simulink model "mixTest123"  (R2020a)
settings: Solver=VariableStepAuto  StartTime=0.0  StopTime=1000  FixedStep=0.05  RelTol=1e-3
InitFcn:
  | data_current
values from neighbouring files (symbols this model uses):
  a1 = rho * D^4 * alpha1    (= 0.000388302366464)    [data_current.m]    (also in main_init.m)
  a2 = -rho * D^3 * alpha2 * (1 - omega)    (= 0.0037030698432)    [data_current.m]    (also in main_init.m)
  ag = [Ax Ay Az]'    [init_modello.m]
  alpha1 = 0.0113    [data_current.m]    (also in main_init.m)
  alpha2 = -0.0091    [data_current.m]    (also in main_init.m)
  areaOfInterestCorner = [42.317744;10.915136; 0]    [init_controllo.m]    (also in missionA.m = [42.317744)
  bg = [Bx By Bz]'    [init_modello.m]
  cd_pitch = 0.7    [init_modello.m]
  cd_roll = 0.04    [init_modello.m]
  cd_x = 0.4    [init_modello.m]
  cd_y = 1    [init_modello.m]
  cd_yaw = 0.7    [init_modello.m]
  cd_z = 1    [init_modello.m]
  cg = [Cx Cy Cz]'    [init_modello.m]
  D = 0.076    [data_current.m]    (also in main_init.m)
  dead_zone_limit = 31.5    [data_current.m]    (also in main_init.m)
  dg = [Dx Dy Dz]'    [init_modello.m]
  eg = [Ex Ey Ez]'    [init_modello.m]
  fg = [Fx Fy Fz]'    [init_modello.m]
  g = 9.81    [init_modello.m]
  galleggiamento = 66.5386    [init_controllo.m]
  gg = [Gx Gy Gz]'    [init_modello.m]
  H0 = 0    [init_modello.m]
  init_position = [pointP(1),pointP(2),0.15,0,0,deg2rad(angle)]'    [appunti.m]    (also in init_modello.m = [pointP(1),pointP(2),0.15,0,0,deg2rad(alpha)]')
  init_velocity = [0 0 0 0 0 0]'    [init_modello.m]
  Ixx = 0.93304097392    [init_modello.m]
  Ixy = 0    [init_modello.m]
  Ixz = 0    [init_modello.m]
  Iyy = 25.58745481378    (= 25.5874548138)    [init_modello.m]
  Iyz = 0    [init_modello.m]
  Izz = 25.58745481378    (= 25.5874548138)    [init_modello.m]
  K_i_heave_div = 20    [init_controllo.m]
  K_i_heave_pos = 1    [init_controllo.m]
  K_i_heave_surf = 20    [init_controllo.m]
  K_i_heave_trans = 5    [init_controllo.m]
  K_i_heave_turn = 5    [init_controllo.m]
  K_i_pitch_div = 0    [init_controllo.m]
  K_i_pitch_pos = 0.1*0    (= 0)    [init_controllo.m]
  K_i_pitch_surf = 0    [init_controllo.m]
  K_i_pitch_trans = 0    [init_controllo.m]
  K_i_pitch_turn = 0    [init_controllo.m]
  K_i_roll_div = 0    [init_controllo.m]
  K_i_roll_pos = 0.1*0    (= 0)    [init_controllo.m]
  K_i_roll_surf = 1    [init_controllo.m]
  K_i_roll_trans = 0    [init_controllo.m]
  K_i_roll_turn = 0    [init_controllo.m]
  K_i_surge_div = 3    [init_controllo.m]
  K_i_surge_pos = 0.1679*30    (= 5.037)    [init_controllo.m]
  K_i_surge_surf = 3    [init_controllo.m]
  K_i_surge_trans = 0.1679*15    (= 2.5185)    [init_controllo.m]
  K_i_surge_turn = 0.1679*60    (= 10.074)    [init_controllo.m]
  K_i_sway_div = 6    [init_controllo.m]
  K_i_sway_pos = 5    [init_controllo.m]
  K_i_sway_surf = 3    [init_controllo.m]
  K_i_sway_trans = 2    [init_controllo.m]
  K_i_sway_turn = 50    [init_controllo.m]
  K_i_yaw_div = 0    [init_controllo.m]
  K_i_yaw_pos = 1    [init_controllo.m]
  K_i_yaw_surf = 0    [init_controllo.m]
  K_i_yaw_trans = 20    [init_controllo.m]
  K_i_yaw_turn = 3    [init_controllo.m]
  K_p_heave_div = 200    [init_controllo.m]
  K_p_heave_pos = 320    [init_controllo.m]
  K_p_heave_surf = 200    [init_controllo.m]
  K_p_heave_trans = 170    [init_controllo.m]
  K_p_heave_turn = 170    [init_controllo.m]
  K_p_phi_div = 0.15    [init_controllo.m]
  K_p_phi_pos = 1*0.1    (= 0.1)    [init_controllo.m]
  K_p_phi_surf = 0.15    [init_controllo.m]
  K_p_phi_trans = 0.1    [init_controllo.m]
  K_p_phi_turn = 0.1    [init_controllo.m]
  K_p_pitch_div = 50    [init_controllo.m]
  K_p_pitch_pos = 25    [init_controllo.m]
  K_p_pitch_surf = 50    [init_controllo.m]
  K_p_pitch_trans = 25    [init_controllo.m]
  K_p_pitch_turn = 25    [init_controllo.m]
  K_p_psi_div = 0.3    [init_controllo.m]
  K_p_psi_pos = 0.25    [init_controllo.m]
  K_p_psi_surf = 0.3    [init_controllo.m]
  K_p_psi_trans = 0.2    [init_controllo.m]
  K_p_roll_div = 10    [init_controllo.m]
  K_p_roll_pos = 0.1*40    (= 4)    [init_controllo.m]
  K_p_roll_surf = 10    [init_controllo.m]
  K_p_roll_trans = 0.1*40    (= 4)    [init_controllo.m]
  K_p_roll_turn = 4    [init_controllo.m]
  K_p_surge_div = 80    [init_controllo.m]
  K_p_surge_pos = 13.7782*2.5    (= 34.4455)    [init_controllo.m]
  K_p_surge_surf = 80    [init_controllo.m]
  K_p_surge_trans = 20    [init_controllo.m]
  K_p_surge_turn = 150    [init_controllo.m]
  K_p_sway_div = 100    [init_controllo.m]
  K_p_sway_pos = 90    [init_controllo.m]
  K_p_sway_surf = 80    [init_controllo.m]
  K_p_sway_trans = 80    [init_controllo.m]
  K_p_sway_turn = 200    [init_controllo.m]
  K_p_th_div = 0.3    [init_controllo.m]
  K_p_th_pos = 0.1    [init_controllo.m]
  K_p_th_surf = 0.3    [init_controllo.m]
  K_p_th_trans = 0.1    [init_controllo.m]
  K_p_th_turn = 0.1    [init_controllo.m]
  K_p_x_div = 0.12    [init_controllo.m]
  K_p_x_pos = 0.12    [init_controllo.m]
  K_p_x_surf = 0.12    [init_controllo.m]
  K_p_y_div = 0.6    [init_controllo.m]
  K_p_y_pos = 0.34    [init_controllo.m]
  K_p_y_surf = 0.1    [init_controllo.m]
  K_p_y_trans = 0.3    [init_controllo.m]
  K_p_y_turn = 0.3    [init_controllo.m]
  K_p_yaw_div = 70    [init_controllo.m]
  K_p_yaw_pos = 20    [init_controllo.m]
  K_p_yaw_surf = 70    [init_controllo.m]
  K_p_yaw_trans = 160    [init_controllo.m]
  K_p_yaw_turn = 60    [init_controllo.m]
  K_p_z_div = 0.35    [init_controllo.m]
  K_p_z_pos = 0.2    [init_controllo.m]
  K_p_z_surf = 0.35    [init_controllo.m]
  K_p_z_trans = 0.10    (= 0.1)    [init_controllo.m]
  K_p_z_turn = 0.1    [init_controllo.m]
  Kadd = 0    [init_modello.m]
  m = 100    [init_modello.m]    (also in retta.m = p2-p1)
  ... (+29 more)
undefined symbols (not defined in the file or in its folder): DiscIntNeverNeededParam
libraries: simulink x4
(part 1 of 5)
settings Model: PauseTimes=1  PacingRate=5  Creator=User  LastModifiedBy=User

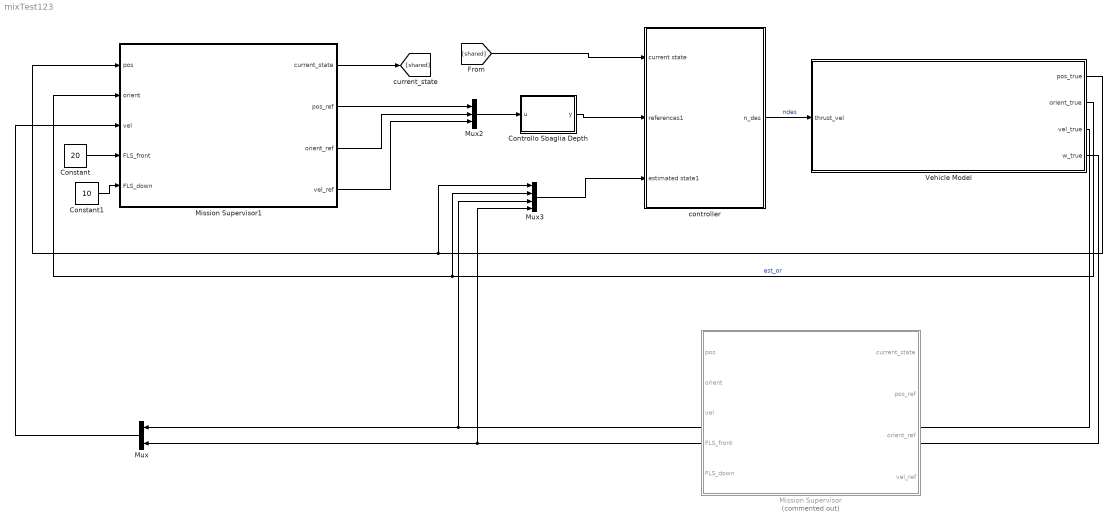
== system mixTest123 ==
  Constant : Constant  Value=20
  Constant1 : Constant  Value=10
  Controllo Sbaglia Depth : MATLAB Function  TreatAsAtomicUnit=on
  Mission Supervisor : Subsystem  Commented=on
  Mission Supervisor1 : Subsystem
  Mux : Mux  Inputs=2
  Mux2 : Mux  Inputs=3
  Mux3 : Mux
  Vehicle Model : Subsystem
  controller : Subsystem
  wires:
  Mission Supervisor1/1(current_state) -> [shared]
  Vehicle Model/3(vel_true) -> Mux3/3, Mux/1
  Vehicle Model/4(w_true) -> Mux3/4, Mux/2
  [shared] -> controller/1(current state)
  Mux2/1 -> Controllo Sbaglia Depth/1(u)
  Mux3/1 -> controller/3(estimated state1)
  controller/1(n_des) -> Vehicle Model/1(thrust_vel)  "ndes"
  Constant/1 -> Mission Supervisor1/4(FLS_front)
  Constant1/1 -> Mission Supervisor1/5(FLS_down)
  Controllo Sbaglia Depth/1(y) -> controller/2(references1)
  Vehicle Model/1(pos_true) -> Mission Supervisor1/1(pos), Mux3/1
  Mission Supervisor1/4(vel_ref) -> Mux2/3
  Vehicle Model/2(orient_true) -> Mission Supervisor1/2(orient), Mux3/2  "est_or"
  Mission Supervisor1/3(orient_ref) -> Mux2/2
  Mux/1 -> Mission Supervisor1/3(vel)
  Mission Supervisor1/2(pos_ref) -> Mux2/1

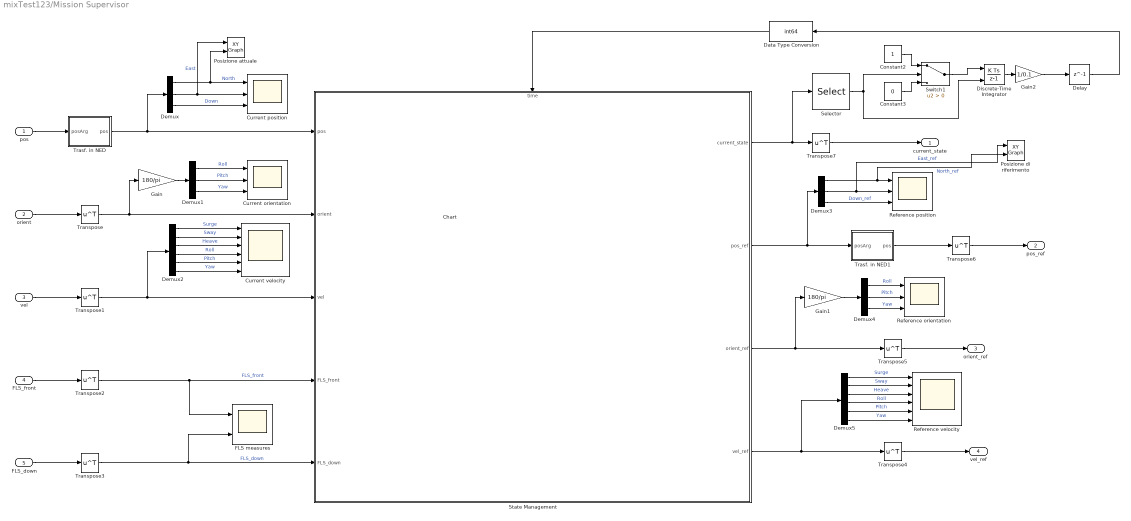
== system mixTest123/Mission Supervisor ==
  pos : Inport
  orient : Inport  Port=2  PortDimensions=[3 1]
  vel : Inport  Port=3  PortDimensions=[6 1]
  FLS_front : Inport  Port=4  PortDimensions=1
  FLS_down : Inport  Port=5  PortDimensions=1
  Chart : Stateflow chart  TreatAsAtomicUnit=on
  Constant2 : Constant
  Constant3 : Constant  Value=0
  Current orientation : Scope  NumInputPorts=3
  Current position : Scope  NumInputPorts=3
  Current velocity : Scope  NumInputPorts=6
  Data Type Conversion : DataTypeConversion  OutDataTypeStr=int64
  Delay : Delay  DelayLength=1  SampleTime=0.1
  Demux{,1,3..4} (4 alike) : Demux  Outputs=3
  Demux2 : Demux  Outputs=6
  Demux5 : Demux  Outputs=6
  Discrete-Time Integrator : DiscreteIntegrator  ExternalReset=falling  SampleTime=0.1  ICPrevOutput=DiscIntNeverNeededParam  ICPrevScaledInput=DiscIntNeverNeededParam
  FLS measures : Scope  NumInputPorts=2
  Gain : Gain  Gain=180/pi
  Gain1 : Gain  Gain=180/pi
  Gain2 : Gain  Gain=1/0.1
  Posizione attuale : simulink/Sinks/XY Graph  xmin=0  xmax=150  ymin=0  ymax=150  st=-1
  Posizione di riferimento : simulink/Sinks/XY Graph  xmin=0  xmax=150  ymin=0  ymax=150  st=-1
  Reference orientation : Scope  NumInputPorts=3
  Reference position : Scope  NumInputPorts=3
  Reference velocity : Scope  NumInputPorts=6
  Selector : Selector  InputPortWidth=8  IndexOptions=Index vector (dialog)  Indices=4  OutputSizes=1
  State Management : Stateflow chart  TreatAsAtomicUnit=on
      settings: PortSchema="{\"entries\":[{\"content\":{\"sides\":[{\"content\":{\"connectorIds\":[\"In1\",\"In2\",\"In3\",\"In4\",\"In5\"]},\"type\":\"ConnectorPlacement.EquallySpacedRectSide\",\"uuid\":\"b4d768e0-b402-4324-9a12-614211dc6b85\"},{\"content\":{\"connectorIds\":[\"Out1\",\"Out2\",\"Out3\",\"Out4\"],\"side\":\"RIGHT\"},\"type\":\"ConnectorPlacement.EquallySpacedRectSide\",\"uuid\":\"64a4c54a-28a4-456f-aa67-ad7da5d6855f\"},{\"content\":{\"connectorIds\":[\"In6\"],\"side\":\"TOP\"},\"type\":\"ConnectorPlacement.EquallySpacedRectSide\",\"uuid\":\"aacc81fd-f61d-4535-bc25-c566f9f9b0ba\"}]},\"type\":\"ConnectorPlacement.EquallySpacedConnector\",\"uuid\":\"1d5bfe1d-6e45-4fc8-afd6-fe82ea6d1d45\"}],\"packageUris\":[\"http://schema.mathworks.com/mf0/Connector/19700101\"],\"version\":\"1.0\"}"
  Switch1 : Switch  Criteria=u2 > Threshold
  Transpose{,1..7} (8 alike) : Math  Operator=transpose  SaturateOnIntegerOverflow=on
  Trasf. in NED : MATLAB Function  TreatAsAtomicUnit=on
  Trasf. in NED1 : MATLAB Function  TreatAsAtomicUnit=on
  current_state : Outport
  pos_ref : Outport  Port=2
  orient_ref : Outport  Port=3
  vel_ref : Outport  Port=4  PortDimensions=[6 1]
  wires:
  Transpose3/1 -> FLS measures/2, State Management/5(FLS_down)  "FLS_down"
  FLS_front/1 -> Transpose2/1
  Transpose5/1 -> orient_ref/1
  orient/1 -> Transpose/1
  vel/1 -> Transpose1/1
  Transpose4/1 -> vel_ref/1
  FLS_down/1 -> Transpose3/1
  Demux/1 -> Posizione attuale/2, Current position/1  "North"
  Demux/2 -> Posizione attuale/1, Current position/2  "East"
  Demux/3 -> Current position/3  "Down"
  Demux1/3 -> Current orientation/3  "Yaw"
  Demux1/2 -> Current orientation/2  "Pitch"
  Transpose/1 -> Gain/1, State Management/2(orient)
  Demux1/1 -> Current orientation/1  "Roll"
  Demux2/1 -> Current velocity/1  "Surge"
  Transpose1/1 -> Demux2/1, State Management/3(vel)
  Demux2/2 -> Current velocity/2  "Sway"
  Demux2/3 -> Current velocity/3  "Heave"
  Transpose2/1 -> FLS measures/1, State Management/4(FLS_front)  "FLS_front"
  Demux2/4 -> Current velocity/4  "Roll"
  Demux2/5 -> Current velocity/5  "Pitch"
  Demux2/6 -> Current velocity/6  "Yaw"
  Demux3/1 -> Posizione di riferimento/2, Reference position/1  "North_ref"
  Demux3/2 -> Posizione di riferimento/1, Reference position/2  "East_ref"
  Demux3/3 -> Reference position/3  "Down_ref"
  Demux4/1 -> Reference orientation/1  "Roll"
  State Management/3(orient_ref) -> Gain1/1, Transpose5/1
  Demux4/2 -> Reference orientation/2  "Pitch"
  Demux4/3 -> Reference orientation/3  "Yaw"
  Demux5/5 -> Reference velocity/5  "Pitch"
  Demux5/2 -> Reference velocity/2  "Sway"
  Demux5/1 -> Reference velocity/1  "Surge"
  Demux5/3 -> Reference velocity/3  "Heave"
  State Management/4(vel_ref) -> Demux5/1, Transpose4/1
  Demux5/4 -> Reference velocity/4  "Roll"
  Demux5/6 -> Reference velocity/6  "Yaw"
  pos/1 -> Trasf. in NED/1(posArg)
  State Management/2(pos_ref) -> Trasf. in NED1/1(posArg), Demux3/1
  Trasf. in NED1/1(pos) -> Transpose6/1
  Trasf. in NED/1(pos) -> Demux/1, State Management/1(pos)
  Transpose6/1 -> pos_ref/1
  Gain/1 -> Demux1/1
  Gain1/1 -> Demux4/1
  Transpose7/1 -> current_state/1
  Discrete-Time Integrator/1 -> Gain2/1
  Selector/1 -> Discrete-Time Integrator/2, Switch1/2
  Switch1/1 -> Discrete-Time Integrator/1
  Constant3/1 -> Switch1/3
  Constant2/1 -> Switch1/1
  Data Type Conversion/1 -> State Management/6(time)
  Gain2/1 -> Delay/1
  Delay/1 -> Data Type Conversion/1
  State Management/1(current_state) -> Selector/1, Transpose7/1

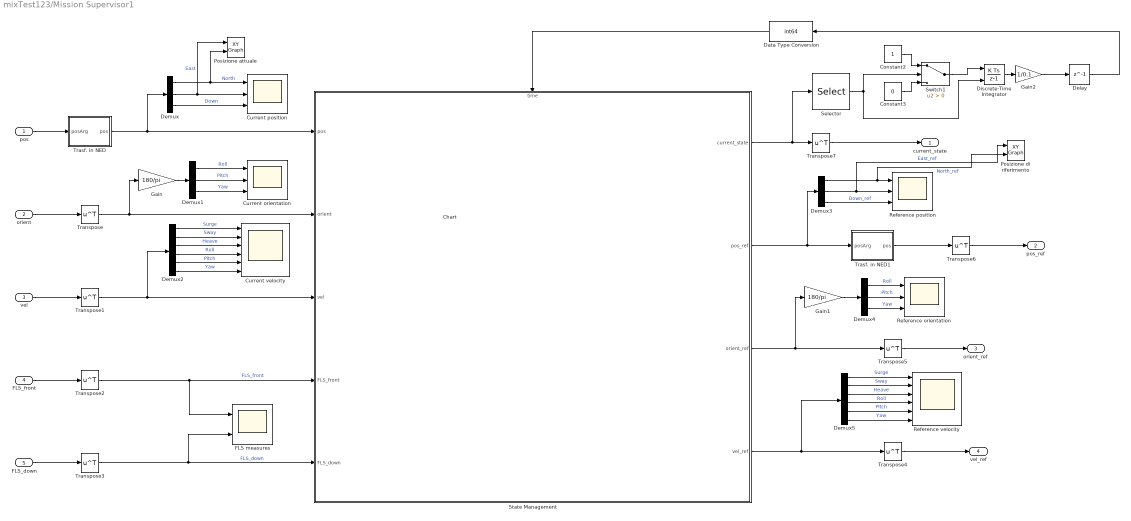
== system mixTest123/Mission Supervisor1 ==
  pos : Inport
  orient : Inport  Port=2  PortDimensions=[3 1]
  vel : Inport  Port=3  PortDimensions=[6 1]
  FLS_front : Inport  Port=4  PortDimensions=1
  FLS_down : Inport  Port=5  PortDimensions=1
  Chart : Stateflow chart  TreatAsAtomicUnit=on
  Constant2 : Constant
  Constant3 : Constant  Value=0
  Current orientation : Scope  NumInputPorts=3
  Current position : Scope  NumInputPorts=3
  Current velocity : Scope  NumInputPorts=6
  Data Type Conversion : DataTypeConversion  OutDataTypeStr=int64
  Delay : Delay  DelayLength=1  SampleTime=0.1
  Demux{,1,3..4} (4 alike) : Demux  Outputs=3
  Demux2 : Demux  Outputs=6
  Demux5 : Demux  Outputs=6
  Discrete-Time Integrator : DiscreteIntegrator  ExternalReset=falling  SampleTime=0.1  ICPrevOutput=DiscIntNeverNeededParam  ICPrevScaledInput=DiscIntNeverNeededParam
  FLS measures : Scope  NumInputPorts=2
  Gain : Gain  Gain=180/pi
  Gain1 : Gain  Gain=180/pi
  Gain2 : Gain  Gain=1/0.1
  Posizione attuale : simulink/Sinks/XY Graph  xmin=0  xmax=150  ymin=0  ymax=150  st=-1
  Posizione di riferimento : simulink/Sinks/XY Graph  xmin=0  xmax=150  ymin=0  ymax=150  st=-1
  Reference orientation : Scope  NumInputPorts=3
  Reference position : Scope  NumInputPorts=3
  Reference velocity : Scope  NumInputPorts=6
  Selector : Selector  InputPortWidth=8  IndexOptions=Index vector (dialog)  Indices=4  OutputSizes=1
  State Management : Stateflow chart  TreatAsAtomicUnit=on
      settings: PortSchema="{\"entries\":[{\"content\":{\"sides\":[{\"content\":{\"connectorIds\":[\"In1\",\"In2\",\"In3\",\"In4\",\"In5\"]},\"type\":\"ConnectorPlacement.EquallySpacedRectSide\",\"uuid\":\"b4d768e0-b402-4324-9a12-614211dc6b85\"},{\"content\":{\"connectorIds\":[\"Out1\",\"Out2\",\"Out3\",\"Out4\"],\"side\":\"RIGHT\"},\"type\":\"ConnectorPlacement.EquallySpacedRectSide\",\"uuid\":\"64a4c54a-28a4-456f-aa67-ad7da5d6855f\"},{\"content\":{\"connectorIds\":[\"In6\"],\"side\":\"TOP\"},\"type\":\"ConnectorPlacement.EquallySpacedRectSide\",\"uuid\":\"aacc81fd-f61d-4535-bc25-c566f9f9b0ba\"}]},\"type\":\"ConnectorPlacement.EquallySpacedConnector\",\"uuid\":\"1d5bfe1d-6e45-4fc8-afd6-fe82ea6d1d45\"}],\"packageUris\":[\"http://schema.mathworks.com/mf0/Connector/19700101\"],\"version\":\"1.0\"}"
  Switch1 : Switch  Criteria=u2 > Threshold
  Transpose{,1..7} (8 alike) : Math  Operator=transpose  SaturateOnIntegerOverflow=on
  Trasf. in NED : MATLAB Function  TreatAsAtomicUnit=on
  Trasf. in NED1 : MATLAB Function  TreatAsAtomicUnit=on
  current_state : Outport
  pos_ref : Outport  Port=2
  orient_ref : Outport  Port=3
  vel_ref : Outport  Port=4  PortDimensions=[6 1]
  wires:
  Transpose3/1 -> FLS measures/2, State Management/5(FLS_down)  "FLS_down"
  FLS_front/1 -> Transpose2/1
  Transpose5/1 -> orient_ref/1
  orient/1 -> Transpose/1
  vel/1 -> Transpose1/1
  Transpose4/1 -> vel_ref/1
  FLS_down/1 -> Transpose3/1
  Demux/1 -> Posizione attuale/2, Current position/1  "North"
  Demux/2 -> Posizione attuale/1, Current position/2  "East"
  Demux/3 -> Current position/3  "Down"
  Demux1/3 -> Current orientation/3  "Yaw"
  Demux1/2 -> Current orientation/2  "Pitch"
  Transpose/1 -> Gain/1, State Management/2(orient)
  Demux1/1 -> Current orientation/1  "Roll"
  Demux2/1 -> Current velocity/1  "Surge"
  Transpose1/1 -> Demux2/1, State Management/3(vel)
  Demux2/2 -> Current velocity/2  "Sway"
  Demux2/3 -> Current velocity/3  "Heave"
  Transpose2/1 -> FLS measures/1, State Management/4(FLS_front)  "FLS_front"
  Demux2/4 -> Current velocity/4  "Roll"
  Demux2/5 -> Current velocity/5  "Pitch"
  Demux2/6 -> Current velocity/6  "Yaw"
  Demux3/1 -> Posizione di riferimento/2, Reference position/1  "North_ref"
  Demux3/2 -> Posizione di riferimento/1, Reference position/2  "East_ref"
  Demux3/3 -> Reference position/3  "Down_ref"
  Demux4/1 -> Reference orientation/1  "Roll"
  State Management/3(orient_ref) -> Gain1/1, Transpose5/1
  Demux4/2 -> Reference orientation/2  "Pitch"
  Demux4/3 -> Reference orientation/3  "Yaw"
  Demux5/5 -> Reference velocity/5  "Pitch"
  Demux5/2 -> Reference velocity/2  "Sway"
  Demux5/1 -> Reference velocity/1  "Surge"
  Demux5/3 -> Reference velocity/3  "Heave"
  State Management/4(vel_ref) -> Demux5/1, Transpose4/1
  Demux5/4 -> Reference velocity/4  "Roll"
  Demux5/6 -> Reference velocity/6  "Yaw"
  pos/1 -> Trasf. in NED/1(posArg)
  State Management/2(pos_ref) -> Trasf. in NED1/1(posArg), Demux3/1
  Trasf. in NED1/1(pos) -> Transpose6/1
  Trasf. in NED/1(pos) -> Demux/1, State Management/1(pos)
  Transpose6/1 -> pos_ref/1
  Gain/1 -> Demux1/1
  Gain1/1 -> Demux4/1
  Transpose7/1 -> current_state/1
  Discrete-Time Integrator/1 -> Gain2/1
  Selector/1 -> Discrete-Time Integrator/2, Switch1/2
  Switch1/1 -> Discrete-Time Integrator/1
  Constant3/1 -> Switch1/3
  Constant2/1 -> Switch1/1
  Data Type Conversion/1 -> State Management/6(time)
  Gain2/1 -> Delay/1
  Delay/1 -> Data Type Conversion/1
  State Management/1(current_state) -> Selector/1, Transpose7/1

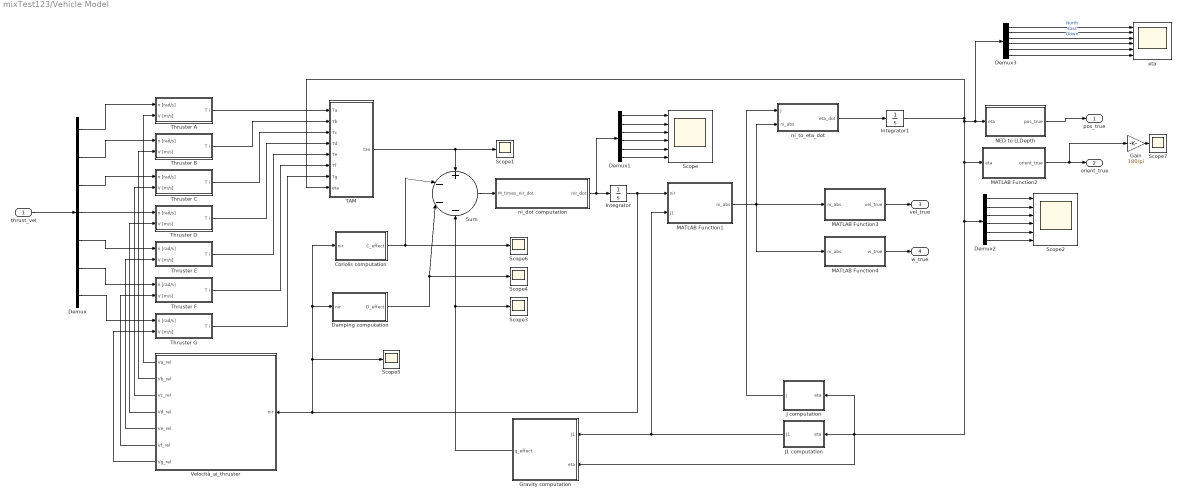
== system mixTest123/Vehicle Model ==
  thrust_vel : Inport
  Coriolis computation : MATLAB Function  TreatAsAtomicUnit=on
  Damping computation : MATLAB Function  TreatAsAtomicUnit=on
  Demux : Demux  Outputs=7
  Demux1 : Demux  Outputs=6
  Demux2 : Demux  Outputs=6
  Demux3 : Demux  Outputs=6
  Gain : Gain  Gain=180/pi
  Gravity computation : MATLAB Function  TreatAsAtomicUnit=on
  Integrator : Integrator  InitialCondition=init_velocity  ContinuousStateAttributes='velocity'
  Integrator1 : Integrator  InitialCondition=init_position  ContinuousStateAttributes='position'
  J computation : MATLAB Function  TreatAsAtomicUnit=on
  J1 computation : MATLAB Function  TreatAsAtomicUnit=on
  MATLAB Function1 : MATLAB Function  TreatAsAtomicUnit=on
  MATLAB Function2 : MATLAB Function  TreatAsAtomicUnit=on
  MATLAB Function3 : MATLAB Function  TreatAsAtomicUnit=on
  MATLAB Function4 : MATLAB Function  TreatAsAtomicUnit=on
  NED to LLDepth : MATLAB Function  TreatAsAtomicUnit=on
  Scope : Scope  NumInputPorts=6
  Scope{1,3..7} (6 alike) : Scope
  Scope2 : Scope  NumInputPorts=6
  Sum : Sum  Inputs=+---
  TAM : MATLAB Function
  Thruster A : Subsystem
  Thruster B : Subsystem
  Thruster C : Subsystem
  Thruster D : Subsystem
  Thruster E : Subsystem
  Thruster F : Subsystem
  Thruster G : Subsystem
  Velocità_ai_thruster : MATLAB Function  TreatAsAtomicUnit=on
  eta : Scope  NumInputPorts=6
  ni_dot computation : MATLAB Function  TreatAsAtomicUnit=on
  ni_to_eta_dot : MATLAB Function  TreatAsAtomicUnit=on
  pos_true : Outport
  orient_true : Outport  Port=2
  vel_true : Outport  Port=3
  w_true : Outport  Port=4
  wires:
  Demux/3 -> Thruster C/1(n [rad/s])
  Thruster A/1(T i) -> TAM/1(Ta)
  Thruster G/1(T i) -> TAM/7(Tg)
  Sum/1 -> ni_dot computation/1(M_times_nir_dot)
  Velocità_ai_thruster/7(Vg_rel) -> Thruster G/2(V [m/s])
  Velocità_ai_thruster/3(Vc_rel) -> Thruster C/2(V [m/s])
  Thruster C/1(T i) -> TAM/3(Tc)
  MATLAB Function3/1(vel_true) -> vel_true/1
  Gravity computation/1(g_effect) -> Sum/4, Scope3/1
  Demux/6 -> Thruster F/1(n [rad/s])
  MATLAB Function4/1(w_true) -> w_true/1
  J1 computation/1(J1) -> Gravity computation/1(J1), MATLAB Function1/2(J1)
  Thruster F/1(T i) -> TAM/6(Tf)
  Integrator/1 -> Scope5/1, Coriolis computation/1(nir), Damping computation/1(nir), Velocità_ai_thruster/1(nir), MATLAB Function1/1(nir)
  Velocità_ai_thruster/4(Vd_rel) -> Thruster D/2(V [m/s])
  Velocità_ai_thruster/6(Vf_rel) -> Thruster F/2(V [m/s])
  ni_dot computation/1(nir_dot) -> Demux1/1, Integrator/1
  Velocità_ai_thruster/2(Vb_rel) -> Thruster B/2(V [m/s])
  MATLAB Function1/1(ni_abs) -> ni_to_eta_dot/2(ni_abs), MATLAB Function3/1(ni_abs), MATLAB Function4/1(ni_abs)
  Velocità_ai_thruster/1(Va_rel) -> Thruster A/2(V [m/s])
  Demux/4 -> Thruster D/1(n [rad/s])
  Thruster E/1(T i) -> TAM/5(Te)
  Thruster B/1(T i) -> TAM/2(Tb)
  Demux/2 -> Thruster B/1(n [rad/s])
  TAM/1(tau) -> Sum/1, Scope1/1
  ni_to_eta_dot/1(eta_dot) -> Integrator1/1
  MATLAB Function2/1(orient_true) -> Gain/1, orient_true/1
  Demux/1 -> Thruster A/1(n [rad/s])
  Velocità_ai_thruster/5(Ve_rel) -> Thruster E/2(V [m/s])
  Demux/5 -> Thruster E/1(n [rad/s])
  NED to LLDepth/1(pos_true) -> pos_true/1
  Thruster D/1(T i) -> TAM/4(Td)
  J computation/1(J) -> ni_to_eta_dot/1(J)
  thrust_vel/1 -> Demux/1
  Demux/7 -> Thruster G/1(n [rad/s])
  Damping computation/1(D_effect) -> Sum/3, Scope4/1
  Coriolis computation/1(C_effect) -> Sum/2, Scope6/1
  Demux1/1 -> Scope/1
  Demux1/2 -> Scope/2
  Demux1/3 -> Scope/3
  Demux1/5 -> Scope/5
  Demux1/6 -> Scope/6
  Demux1/4 -> Scope/4
  Demux2/6 -> Scope2/6
  Demux2/5 -> Scope2/5
  Demux2/3 -> Scope2/3
  Demux2/2 -> Scope2/2
  Demux2/4 -> Scope2/4
  Demux2/1 -> Scope2/1
  Demux3/3 -> eta/3  "Down"
  Demux3/1 -> eta/1  "North"
  Demux3/2 -> eta/2  "East"
  Integrator1/1 -> TAM/8(eta), Demux3/1, NED to LLDepth/1(eta), J computation/1(eta), Gravity computation/2(eta), J1 computation/1(eta), Demux2/1, MATLAB Function2/1(eta)
  Demux3/4 -> eta/4
  Demux3/5 -> eta/5
  Demux3/6 -> eta/6
  Gain/1 -> Scope7/1

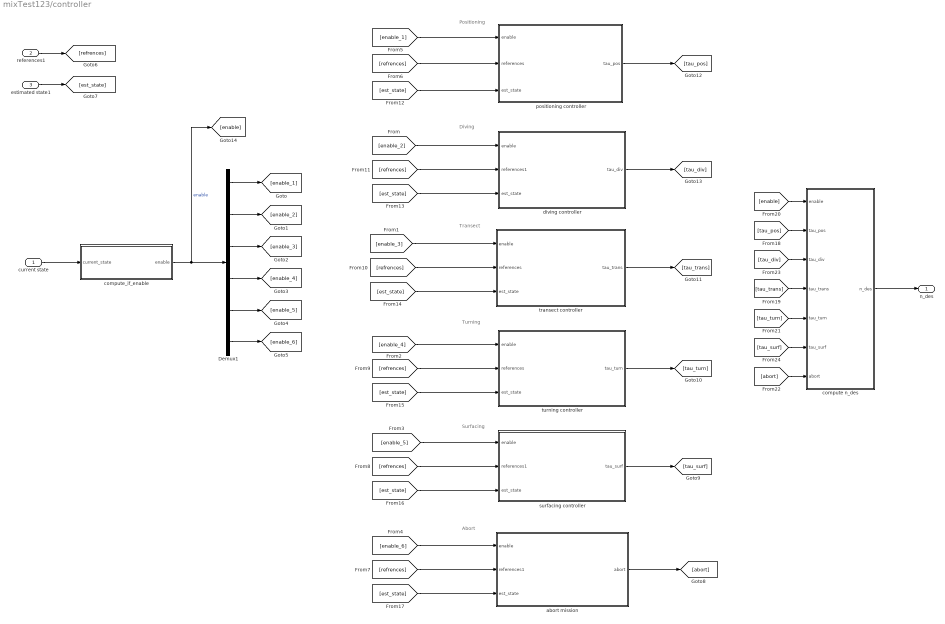
== system mixTest123/controller ==
  note: Diving
  note: Positioning
  note: Transect
  note: Abort
  note: Surfacing
  note: Turning
  current state : Inport
  references1 : Inport  Port=2
  estimated state1 : Inport  Port=3
  Demux1 : Demux  Outputs=6
  abort mission : Subsystem
  compute n_des : MATLAB Function  TreatAsAtomicUnit=on
  compute_if_enable : MATLAB Function  TreatAsAtomicUnit=on
  diving controller : Subsystem
  positioning controller : Subsystem
  surfacing controller : Subsystem
  transect controller : Subsystem
  turning controller : Subsystem
  n_des : Outport
  wires:
  [enable] -> compute n_des/1(enable)
  [enable_5] -> surfacing controller/1(enable)
  abort mission/1(abort) -> [abort]
  compute_if_enable/1(enable) -> [enable], Demux1/1  "enable"
  Demux1/3 -> [enable_3]
  Demux1/4 -> [enable_4]
  [tau_pos] -> compute n_des/2(tau_pos)
  [tau_surf] -> compute n_des/6(tau_surf)
  Demux1/5 -> [enable_5]
  Demux1/6 -> [enable_6]
  [refrences] -> diving controller/2(references1)
  references1/1 -> [refrences]
  turning controller/1(tau_turn) -> [tau_turn]
  [enable_2] -> diving controller/1(enable)
  [enable_4] -> turning controller/1(enable)
  [est_state] -> abort mission/3(est_state)
  current state/1 -> compute_if_enable/1(current_state)
  [tau_turn] -> compute n_des/5(tau_turn)
  [enable_1] -> positioning controller/1(enable)
  [refrences] -> abort mission/2(references1)
  Demux1/2 -> [enable_2]
  [est_state] -> turning controller/3(est_state)
  Demux1/1 -> [enable_1]
  [refrences] -> transect controller/2(references)
  diving controller/1(tau_div) -> [tau_div]
  [tau_trans] -> compute n_des/4(tau_trans)
  positioning controller/1(tau_pos) -> [tau_pos]
  [tau_div] -> compute n_des/3(tau_div)
  surfacing controller/1(tau_surf) -> [tau_surf]
  [abort] -> compute n_des/7(abort)
  [refrences] -> surfacing controller/2(references1)
  [enable_3] -> transect controller/1(enable)
  [refrences] -> positioning controller/2(references)
  [refrences] -> turning controller/2(references)
  [enable_6] -> abort mission/1(enable)
  estimated state1/1 -> [est_state]
  [est_state] -> positioning controller/3(est_state)
  [est_state] -> diving controller/3(est_state)
  transect controller/1(tau_trans) -> [tau_trans]
  [est_state] -> transect controller/3(est_state)
  [est_state] -> surfacing controller/3(est_state)
  compute n_des/1(n_des) -> n_des/1

== system mixTest123/Mission Supervisor/State Management/Movements.End ==
  f : TriggerPort  TriggerType=function-call  VariantControl=(inherit)
      settings: CopyFcn=Stateflow.SLINSF.SimulinkMan.removeBlockPreDeleteFcn  PreDeleteFcn=Stateflow.SLINSF.SimulinkMan.unsafePredeleteFcn
  Constant : Constant
  Stop Simulation : Stop
  wires:
  Constant/1 -> Stop Simulation/1

== system mixTest123/Mission Supervisor1/State Management/Movements.End ==
  f : TriggerPort  TriggerType=function-call  VariantControl=(inherit)
      settings: CopyFcn=Stateflow.SLINSF.SimulinkMan.removeBlockPreDeleteFcn  PreDeleteFcn=Stateflow.SLINSF.SimulinkMan.unsafePredeleteFcn
  Constant : Constant
  Stop Simulation : Stop
  wires:
  Constant/1 -> Stop Simulation/1

== system mixTest123/Vehicle Model/Thruster A ==
  note: n is the rotational speed of the thruster
      | V is the speed component of the water along the thruster axis
      |
      | n is saturated according to data
      | a dead zone is considered according to data
      | the thruster is characterised by 1st order dynamics (tau = 0.2s)
  n [rad/s] : Inport
  V [m/s] : Inport  Port=2
  Dead Zone : DeadZone  LowerValue=-dead_zone_limit  UpperValue=dead_zone_limit  SaturateOnIntegerOverflow=on
  MATLAB Function : MATLAB Function  TreatAsAtomicUnit=on
  Saturation : Saturate  UpperLimit=n_max  LowerLimit=-n_max
  Transfer Fcn : TransferFcn  Denominator=[0.2 1]
  T i : Outport
  wires:
  V [m/s]/1 -> MATLAB Function/2(V)
  Saturation/1 -> MATLAB Function/1(n)
  Transfer Fcn/1 -> Saturation/1
  Dead Zone/1 -> Transfer Fcn/1
  n [rad/s]/1 -> Dead Zone/1
  MATLAB Function/1(T) -> T i/1

== system mixTest123/Vehicle Model/Thruster B ==
  note: n is the rotational speed of the thruster
      | V is the speed component of the water along the thruster axis
      |
      | n is saturated according to data
      | a dead zone is considered according to data
      | the thruster is characterised by 1st order dynamics (tau = 0.2s)
  n [rad/s] : Inport
  V [m/s] : Inport  Port=2
  Dead Zone : DeadZone  LowerValue=-dead_zone_limit  UpperValue=dead_zone_limit  SaturateOnIntegerOverflow=on
  MATLAB Function : MATLAB Function  TreatAsAtomicUnit=on
  Saturation : Saturate  UpperLimit=n_max  LowerLimit=-n_max
  Transfer Fcn : TransferFcn  Denominator=[0.2 1]
  T i : Outport
  wires:
  MATLAB Function/1(T) -> T i/1
  n [rad/s]/1 -> Dead Zone/1
  Dead Zone/1 -> Transfer Fcn/1
  Transfer Fcn/1 -> Saturation/1
  Saturation/1 -> MATLAB Function/1(n)
  V [m/s]/1 -> MATLAB Function/2(V)

== system mixTest123/Vehicle Model/Thruster C ==
  note: n is the rotational speed of the thruster
      | V is the speed component of the water along the thruster axis
      |
      | n is saturated according to data
      | a dead zone is considered according to data
      | the thruster is characterised by 1st order dynamics (tau = 0.2s)
  n [rad/s] : Inport
  V [m/s] : Inport  Port=2
  Dead Zone : DeadZone  LowerValue=-dead_zone_limit  UpperValue=dead_zone_limit  SaturateOnIntegerOverflow=on
  MATLAB Function : MATLAB Function  TreatAsAtomicUnit=on
  Saturation : Saturate  UpperLimit=n_max  LowerLimit=-n_max
  Transfer Fcn : TransferFcn  Denominator=[0.2 1]
  T i : Outport
  wires:
  V [m/s]/1 -> MATLAB Function/2(V)
  Saturation/1 -> MATLAB Function/1(n)
  Transfer Fcn/1 -> Saturation/1
  Dead Zone/1 -> Transfer Fcn/1
  n [rad/s]/1 -> Dead Zone/1
  MATLAB Function/1(T) -> T i/1

== system mixTest123/Vehicle Model/Thruster D ==
  note: n is the rotational speed of the thruster
      | V is the speed component of the water along the thruster axis
      |
      | n is saturated according to data
      | a dead zone is considered according to data
      | the thruster is characterised by 1st order dynamics (tau = 0.2s)
  n [rad/s] : Inport
  V [m/s] : Inport  Port=2
  Dead Zone : DeadZone  LowerValue=-dead_zone_limit  UpperValue=dead_zone_limit  SaturateOnIntegerOverflow=on
  MATLAB Function : MATLAB Function  TreatAsAtomicUnit=on
  Saturation : Saturate  UpperLimit=n_max  LowerLimit=-n_max
  Transfer Fcn : TransferFcn  Denominator=[0.2 1]
  T i : Outport
  wires:
  MATLAB Function/1(T) -> T i/1
  n [rad/s]/1 -> Dead Zone/1
  Dead Zone/1 -> Transfer Fcn/1
  Transfer Fcn/1 -> Saturation/1
  Saturation/1 -> MATLAB Function/1(n)
  V [m/s]/1 -> MATLAB Function/2(V)

== system mixTest123/Vehicle Model/Thruster E ==
  note: n is the rotational speed of the thruster
      | V is the speed component of the water along the thruster axis
      |
      | n is saturated according to data
      | a dead zone is considered according to data
      | the thruster is characterised by 1st order dynamics (tau = 0.2s)
  n [rad/s] : Inport
  V [m/s] : Inport  Port=2
  Dead Zone : DeadZone  LowerValue=-dead_zone_limit  UpperValue=dead_zone_limit  SaturateOnIntegerOverflow=on
  MATLAB Function : MATLAB Function  TreatAsAtomicUnit=on
  Saturation : Saturate  UpperLimit=n_max  LowerLimit=-n_max
  Transfer Fcn : TransferFcn  Denominator=[0.2 1]
  T i : Outport
  wires:
  V [m/s]/1 -> MATLAB Function/2(V)
  Saturation/1 -> MATLAB Function/1(n)
  Transfer Fcn/1 -> Saturation/1
  Dead Zone/1 -> Transfer Fcn/1
  n [rad/s]/1 -> Dead Zone/1
  MATLAB Function/1(T) -> T i/1

== system mixTest123/Vehicle Model/Thruster F ==
  note: n is the rotational speed of the thruster
      | V is the speed component of the water along the thruster axis
      |
      | n is saturated according to data
      | a dead zone is considered according to data
      | the thruster is characterised by 1st order dynamics (tau = 0.2s)
  n [rad/s] : Inport
  V [m/s] : Inport  Port=2
  Dead Zone : DeadZone  LowerValue=-dead_zone_limit  UpperValue=dead_zone_limit  SaturateOnIntegerOverflow=on
  MATLAB Function : MATLAB Function  TreatAsAtomicUnit=on
  Saturation : Saturate  UpperLimit=n_max  LowerLimit=-n_max
  Transfer Fcn : TransferFcn  Denominator=[0.2 1]
  T i : Outport
  wires:
  MATLAB Function/1(T) -> T i/1
  n [rad/s]/1 -> Dead Zone/1
  Dead Zone/1 -> Transfer Fcn/1
  Transfer Fcn/1 -> Saturation/1
  Saturation/1 -> MATLAB Function/1(n)
  V [m/s]/1 -> MATLAB Function/2(V)

== system mixTest123/Vehicle Model/Thruster G ==
  note: n is the rotational speed of the thruster
      | V is the speed component of the water along the thruster axis
      |
      | n is saturated according to data
      | a dead zone is considered according to data
      | the thruster is characterised by 1st order dynamics (tau = 0.2s)
  n [rad/s] : Inport
  V [m/s] : Inport  Port=2
  Dead Zone : DeadZone  LowerValue=-dead_zone_limit  UpperValue=dead_zone_limit  SaturateOnIntegerOverflow=on
  MATLAB Function : MATLAB Function  TreatAsAtomicUnit=on
  Saturation : Saturate  UpperLimit=n_max  LowerLimit=-n_max
  Transfer Fcn : TransferFcn  Denominator=[0.2 1]
  T i : Outport
  wires:
  V [m/s]/1 -> MATLAB Function/2(V)
  Saturation/1 -> MATLAB Function/1(n)
  Transfer Fcn/1 -> Saturation/1
  Dead Zone/1 -> Transfer Fcn/1
  n [rad/s]/1 -> Dead Zone/1
  MATLAB Function/1(T) -> T i/1

== system mixTest123/controller/abort mission ==
  enable : Inport
  references1 : Inport  Port=2
  est_state : Inport  Port=3
  abort mission : MATLAB Function  TreatAsAtomicUnit=on
  abort : Outport
  wires:
  enable/1 -> abort mission/1(enable)
  references1/1 -> abort mission/2(ref)
  est_state/1 -> abort mission/3(est_meas)
  abort mission/1(abort) -> abort/1

== system mixTest123/controller/diving controller ==
  enable : Inport
  references1 : Inport  Port=2
  est_state : Inport  Port=3
  Mux : Mux  Inputs=6
  heave_controller : Subsystem
  pitch_controller : Subsystem
  roll_controller : Subsystem
  surge_controller : Subsystem
  sway_controller : Subsystem
  yaw_controller : Subsystem
  tau_div : Outport
  wires:
  sway_controller/1(Y) -> Mux/2  "Y"
  yaw_controller/1(N) -> Mux/6  "N"
  Mux/1 -> tau_div/1
  heave_controller/1(Z) -> Mux/3  "Z"
  references1/1 -> surge_controller/2(references), heave_controller/2(references), roll_controller/2(references), yaw_controller/2(references), pitch_controller/2(references), sway_controller/2(references)
  est_state/1 -> sway_controller/3("estimated measures "), heave_controller/3("estimated measures "), roll_controller/3("estimated measures "), yaw_controller/3("estimated measures "), pitch_controller/3("estimated measures "), surge_controller/3("estimated measures ")
  surge_controller/1(X) -> Mux/1  "X"
  roll_controller/1(K) -> Mux/4  "K"
  pitch_controller/1(M) -> Mux/5  "M"
  enable/1 -> sway_controller/1(enable), heave_controller/1(enable), yaw_controller/1(enable), pitch_controller/1(enable), roll_controller/1(enable), surge_controller/1(enable)

== system mixTest123/controller/positioning controller ==
  enable : Inport
  references : Inport  Port=2
  est_state : Inport  Port=3
  Mux : Mux  Inputs=6
  heave_controller : Subsystem
  pitch_controller : Subsystem
  roll_controller : Subsystem
  surge_controller : Subsystem
  sway_controller : Subsystem
  yaw_controller : Subsystem
  tau_pos : Outport
  wires:
  enable/1 -> sway_controller/1(enable), heave_controller/1(enable), yaw_controller/1(enable), pitch_controller/1(enable), roll_controller/1(enable), surge_controller/1(enable)
  yaw_controller/1(N) -> Mux/6  "N"
  references/1 -> surge_controller/2(references), heave_controller/2(references), roll_controller/2(references), yaw_controller/2(references), pitch_controller/2(references), sway_controller/2(references)
  pitch_controller/1(M) -> Mux/5  "M"
  est_state/1 -> sway_controller/3("estimated measures "), heave_controller/3("estimated measures "), roll_controller/3("estimated measures "), yaw_controller/3("estimated measures "), pitch_controller/3("estimated measures "), surge_controller/3("estimated measures ")
  surge_controller/1(X) -> Mux/1  "X"
  sway_controller/1(Y) -> Mux/2  "Y"
  roll_controller/1(K) -> Mux/4  "K"
  Mux/1 -> tau_pos/1
  heave_controller/1(Z) -> Mux/3  "Z"

== system mixTest123/controller/surfacing controller ==
  enable : Inport
  references1 : Inport  Port=2
  est_state : Inport  Port=3
  Mux : Mux  Inputs=6
  heave_controller : Subsystem
  pitch_controller : Subsystem
  roll_controller : Subsystem
  surge_controller : Subsystem
  sway_controller : Subsystem
  yaw_controller : Subsystem
  tau_surf : Outport
  wires:
  sway_controller/1(Y) -> Mux/2  "Y"
  yaw_controller/1(N) -> Mux/6  "N"
  Mux/1 -> tau_surf/1
  heave_controller/1(Z) -> Mux/3  "Z"
  references1/1 -> surge_controller/2(references), heave_controller/2(references), roll_controller/2(references), yaw_controller/2(references), pitch_controller/2(references), sway_controller/2(references)
  est_state/1 -> sway_controller/3("estimated measures "), heave_controller/3("estimated measures "), roll_controller/3("estimated measures "), yaw_controller/3("estimated measures "), pitch_controller/3("estimated measures "), surge_controller/3("estimated measures ")
  surge_controller/1(X) -> Mux/1  "X"
  roll_controller/1(K) -> Mux/4  "K"
  pitch_controller/1(M) -> Mux/5  "M"
  enable/1 -> sway_controller/1(enable), heave_controller/1(enable), yaw_controller/1(enable), pitch_controller/1(enable), roll_controller/1(enable), surge_controller/1(enable)

== system mixTest123/controller/transect controller ==
  enable : Inport
  references : Inport  Port=2
  est_state : Inport  Port=3
  Mux : Mux  Inputs=6
  heave_controller : Subsystem
  pitch_controller : Subsystem
  roll_controller : Subsystem
  surge_controller : Subsystem
  sway_controller : Subsystem
  yaw_controller : Subsystem
  tau_trans : Outport
  wires:
  sway_controller/1(Y) -> Mux/2  "Y"
  yaw_controller/1(N) -> Mux/6  "N"
  Mux/1 -> tau_trans/1
  heave_controller/1(Z) -> Mux/3  "Z"
  references/1 -> surge_controller/2(references), heave_controller/2(references), roll_controller/2(references), yaw_controller/2(references), pitch_controller/2(references), sway_controller/2(references)
  est_state/1 -> sway_controller/3("estimated measures "), heave_controller/3("estimated measures "), roll_controller/3("estimated measures "), yaw_controller/3("estimated measures "), pitch_controller/3("estimated measures "), surge_controller/3("estimated measures ")
  surge_controller/1(X) -> Mux/1  "X"
  roll_controller/1(K) -> Mux/4  "K"
  pitch_controller/1(M) -> Mux/5  "M"
  enable/1 -> sway_controller/1(enable), heave_controller/1(enable), yaw_controller/1(enable), pitch_controller/1(enable), roll_controller/1(enable), surge_controller/1(enable)

== system mixTest123/controller/turning controller ==
  enable : Inport
  references : Inport  Port=2
  est_state : Inport  Port=3
  Mux : Mux  Inputs=6
  heave_controller : Subsystem
  pitch_controller : Subsystem
  roll_controller : Subsystem
  surge_controller : Subsystem
  sway_controller : Subsystem
  yaw_controller : Subsystem
  tau_turn : Outport
  wires:
  sway_controller/1(Y) -> Mux/2  "Y"
  yaw_controller/1(N) -> Mux/6  "N"
  Mux/1 -> tau_turn/1
  heave_controller/1(Z) -> Mux/3  "Z"
  references/1 -> surge_controller/2(references), heave_controller/2(references), roll_controller/2(references), yaw_controller/2(references), pitch_controller/2(references), sway_controller/2(references)
  est_state/1 -> sway_controller/3("estimated measures "), heave_controller/3("estimated measures "), roll_controller/3("estimated measures "), yaw_controller/3("estimated measures "), pitch_controller/3("estimated measures "), surge_controller/3("estimated measures ")
  surge_controller/1(X) -> Mux/1  "X"
  roll_controller/1(K) -> Mux/4  "K"
  pitch_controller/1(M) -> Mux/5  "M"
  enable/1 -> sway_controller/1(enable), heave_controller/1(enable), yaw_controller/1(enable), pitch_controller/1(enable), roll_controller/1(enable), surge_controller/1(enable)

== system mixTest123/controller/diving controller/heave_controller ==
  enable : Inport
  references : Inport  Port=2
  "estimated measures " : Inport  Port=3
  Heave PID controller : Subsystem
  Z : Outport
  wires:
  Heave PID controller/1(Z) -> Z/1  "Z_pid"
  references/1 -> Heave PID controller/2(references)
  enable/1 -> Heave PID controller/1(enable)
  "estimated measures "/1 -> Heave PID controller/3("estimated measures ")

== system mixTest123/controller/diving controller/pitch_controller ==
  enable : Inport
  references : Inport  Port=2
  "estimated measures " : Inport  Port=3
  Pitch PID controller : Subsystem
  M : Outport
  wires:
  enable/1 -> Pitch PID controller/1(enable)
  "estimated measures "/1 -> Pitch PID controller/3("estimated measures ")
  references/1 -> Pitch PID controller/2(references)
  Pitch PID controller/1(tau_pitch) -> M/1  "M_pid"

== system mixTest123/controller/diving controller/roll_controller ==
  enable : Inport
  references : Inport  Port=2
  "estimated measures " : Inport  Port=3
  Roll PID controller : Subsystem
  K : Outport
  wires:
  "estimated measures "/1 -> Roll PID controller/3("estimated measures ")
  Roll PID controller/1(tau_roll) -> K/1  "K_pid"
  references/1 -> Roll PID controller/2(references)
  enable/1 -> Roll PID controller/1(enable)

== system mixTest123/controller/diving controller/surge_controller ==
  enable : Inport
  references : Inport  Port=2
  "estimated measures " : Inport  Port=3
  Surge PID controller : Subsystem
  X : Outport
  wires:
  references/1 -> Surge PID controller/2(references)
  "estimated measures "/1 -> Surge PID controller/3("estimated measures ")
  Surge PID controller/1(X) -> X/1  "X_pid"
  enable/1 -> Surge PID controller/1(enable)

== system mixTest123/controller/diving controller/sway_controller ==
  enable : Inport
  references : Inport  Port=2
  "estimated measures " : Inport  Port=3
  Sway PID controller : Subsystem
  Y : Outport
  wires:
  enable/1 -> Sway PID controller/1(enable)
  "estimated measures "/1 -> Sway PID controller/3("estimated measures ")
  references/1 -> Sway PID controller/2(references)
  Sway PID controller/1(Y) -> Y/1  "Y_pid"

== system mixTest123/controller/diving controller/yaw_controller ==
  enable : Inport
  references : Inport  Port=2
  "estimated measures " : Inport  Port=3
  Yaw PID controller : Subsystem
  N : Outport
  wires:
  enable/1 -> Yaw PID controller/1(enable)
  "estimated measures "/1 -> Yaw PID controller/3("estimated measures ")
  references/1 -> Yaw PID controller/2(references)
  Yaw PID controller/1(tau_yaw) -> N/1  "N_pid"

== system mixTest123/controller/positioning controller/heave_controller ==
  enable : Inport
  references : Inport  Port=2
  "estimated measures " : Inport  Port=3
  Heave PID controller : Subsystem
  Z : Outport
  wires:
  Heave PID controller/1(Z) -> Z/1  "Z_pid"
  references/1 -> Heave PID controller/2(references)  "ref"
  enable/1 -> Heave PID controller/1(enable)
  "estimated measures "/1 -> Heave PID controller/3("estimated measures ")  "est_meas"

== system mixTest123/controller/positioning controller/pitch_controller ==
  enable : Inport
  references : Inport  Port=2
  "estimated measures " : Inport  Port=3
  Pitch PID controller : Subsystem
  M : Outport
  wires:
  enable/1 -> Pitch PID controller/1(enable)
  "estimated measures "/1 -> Pitch PID controller/3("estimated measures ")
  references/1 -> Pitch PID controller/2(references)
  Pitch PID controller/1(tau_pitch) -> M/1  "M_pid"

== system mixTest123/controller/positioning controller/roll_controller ==
  enable : Inport
  references : Inport  Port=2
  "estimated measures " : Inport  Port=3
  Roll PID controller : Subsystem
  K : Outport
  wires:
  "estimated measures "/1 -> Roll PID controller/3("estimated measures ")
  Roll PID controller/1(tau_roll) -> K/1  "K_pid"
  references/1 -> Roll PID controller/2(references)
  enable/1 -> Roll PID controller/1(enable)

== system mixTest123/controller/positioning controller/surge_controller ==
  enable : Inport
  references : Inport  Port=2
  "estimated measures " : Inport  Port=3
  Surge PID controller : Subsystem
  X : Outport
  wires:
  references/1 -> Surge PID controller/2(references)  "ref"
  "estimated measures "/1 -> Surge PID controller/3("estimated measures ")  "est_meas"
  Surge PID controller/1(X) -> X/1  "X_pid"
  enable/1 -> Surge PID controller/1(enable)

== system mixTest123/controller/positioning controller/sway_controller ==
  enable : Inport
  references : Inport  Port=2
  "estimated measures " : Inport  Port=3
  Sway PID controller : Subsystem
  Y : Outport
  wires:
  enable/1 -> Sway PID controller/1(enable)
  "estimated measures "/1 -> Sway PID controller/3("estimated measures ")
  references/1 -> Sway PID controller/2(references)
  Sway PID controller/1(Y) -> Y/1  "Y_pid"

== system mixTest123/controller/positioning controller/yaw_controller ==
  enable : Inport
  references : Inport  Port=2
  "estimated measures " : Inport  Port=3
  Yaw PID controller : Subsystem
  N : Outport
  wires:
  enable/1 -> Yaw PID controller/1(enable)
  "estimated measures "/1 -> Yaw PID controller/3("estimated measures ")  "est_meas"
  references/1 -> Yaw PID controller/2(references)  "ref"
  Yaw PID controller/1(tau_yaw) -> N/1  "N_pid"

== system mixTest123/controller/surfacing controller/heave_controller ==
  enable : Inport
  references : Inport  Port=2
  "estimated measures " : Inport  Port=3
  Heave PID controller : Subsystem
  Z : Outport
  wires:
  Heave PID controller/1(Z) -> Z/1  "Z_pid"
  references/1 -> Heave PID controller/2(references)
  enable/1 -> Heave PID controller/1(enable)
  "estimated measures "/1 -> Heave PID controller/3("estimated measures ")

== system mixTest123/controller/surfacing controller/pitch_controller ==
  enable : Inport
  references : Inport  Port=2
  "estimated measures " : Inport  Port=3
  Pitch PID controller : Subsystem
  M : Outport
  wires:
  enable/1 -> Pitch PID controller/1(enable)
  "estimated measures "/1 -> Pitch PID controller/3("estimated measures ")
  references/1 -> Pitch PID controller/2(references)
  Pitch PID controller/1(M) -> M/1  "M_pid"

== system mixTest123/controller/surfacing controller/roll_controller ==
  enable : Inport
  references : Inport  Port=2
  "estimated measures " : Inport  Port=3
  Roll PID controller : Subsystem
  K : Outport
  wires:
  "estimated measures "/1 -> Roll PID controller/3("estimated measures ")
  Roll PID controller/1(K) -> K/1  "K_pid"
  references/1 -> Roll PID controller/2(references)
  enable/1 -> Roll PID controller/1(enable)

== system mixTest123/controller/surfacing controller/surge_controller ==
  enable : Inport
  references : Inport  Port=2
  "estimated measures " : Inport  Port=3
  Surge PID controller : Subsystem
  X : Outport
  wires:
  references/1 -> Surge PID controller/2(references)
  "estimated measures "/1 -> Surge PID controller/3("estimated measures ")
  Surge PID controller/1(X) -> X/1  "X_pid"
  enable/1 -> Surge PID controller/1(enable)

== system mixTest123/controller/surfacing controller/sway_controller ==
  enable : Inport
  references : Inport  Port=2
  "estimated measures " : Inport  Port=3
  Sway PID controller : Subsystem
  Y : Outport
  wires:
  enable/1 -> Sway PID controller/1(enable)
  "estimated measures "/1 -> Sway PID controller/3("estimated measures ")
  references/1 -> Sway PID controller/2(references)
  Sway PID controller/1(Y) -> Y/1  "Y_pid"

== system mixTest123/controller/surfacing controller/yaw_controller ==
  enable : Inport
  references : Inport  Port=2
  "estimated measures " : Inport  Port=3
  Yaw PID controller : Subsystem
  N : Outport
  wires:
  enable/1 -> Yaw PID controller/1(enable)
  "estimated measures "/1 -> Yaw PID controller/3("estimated measures ")
  references/1 -> Yaw PID controller/2(references)
  Yaw PID controller/1(N) -> N/1  "N_pid"

== system mixTest123/controller/transect controller/heave_controller ==
  enable : Inport
  references : Inport  Port=2
  "estimated measures " : Inport  Port=3
  Heave PID controller : Subsystem
  Z : Outport
  wires:
  Heave PID controller/1(Z) -> Z/1  "Z_pid"
  references/1 -> Heave PID controller/2(references)
  enable/1 -> Heave PID controller/1(enable)
  "estimated measures "/1 -> Heave PID controller/3("estimated measures ")

== system mixTest123/controller/transect controller/pitch_controller ==
  enable : Inport
  references : Inport  Port=2
  "estimated measures " : Inport  Port=3
  Pitch PID controller : Subsystem
  M : Outport
  wires:
  enable/1 -> Pitch PID controller/1(enable)
  "estimated measures "/1 -> Pitch PID controller/3("estimated measures ")
  references/1 -> Pitch PID controller/2(references)
  Pitch PID controller/1(M) -> M/1  "M_pid"

== system mixTest123/controller/transect controller/roll_controller ==
  enable : Inport
  references : Inport  Port=2
  "estimated measures " : Inport  Port=3
  Roll PID controller : Subsystem
  K : Outport
  wires:
  "estimated measures "/1 -> Roll PID controller/3("estimated measures ")
  Roll PID controller/1(tau_roll) -> K/1  "K_pid"
  references/1 -> Roll PID controller/2(references)
  enable/1 -> Roll PID controller/1(enable)

== system mixTest123/controller/transect controller/surge_controller ==
  enable : Inport
  references : Inport  Port=2
  "estimated measures " : Inport  Port=3
  Surge PID controller : Subsystem
  X : Outport
  wires:
  references/1 -> Surge PID controller/2(ref)
  "estimated measures "/1 -> Surge PID controller/3(est_meas)
  Surge PID controller/1(X) -> X/1  "X_pid"
  enable/1 -> Surge PID controller/1(enable)

== system mixTest123/controller/transect controller/sway_controller ==
  enable : Inport
  references : Inport  Port=2
  "estimated measures " : Inport  Port=3
  Sway PID controller : Subsystem
  Y : Outport
  wires:
  enable/1 -> Sway PID controller/1(enable)
  "estimated measures "/1 -> Sway PID controller/3("estimated measures ")
  references/1 -> Sway PID controller/2(references)
  Sway PID controller/1(Y) -> Y/1  "Y_pid"

== system mixTest123/controller/transect controller/yaw_controller ==
  enable : Inport
  references : Inport  Port=2
  "estimated measures " : Inport  Port=3
  Yaw PID controller : Subsystem
  N : Outport
  wires:
  enable/1 -> Yaw PID controller/1(enable)
  "estimated measures "/1 -> Yaw PID controller/3("estimated measures ")
  references/1 -> Yaw PID controller/2(references)
  Yaw PID controller/1(N) -> N/1  "N_pid"

== system mixTest123/controller/turning controller/heave_controller ==
  enable : Inport
  references : Inport  Port=2
  "estimated measures " : Inport  Port=3
  Heave PID controller : Subsystem
  Z : Outport
  wires:
  Heave PID controller/1(Z) -> Z/1  "Z_pid"
  references/1 -> Heave PID controller/2(references)
  enable/1 -> Heave PID controller/1(enable)
  "estimated measures "/1 -> Heave PID controller/3("estimated measures ")

== system mixTest123/controller/turning controller/pitch_controller ==
  enable : Inport
  references : Inport  Port=2
  "estimated measures " : Inport  Port=3
  Pitch PID controller : Subsystem
  M : Outport
  wires:
  enable/1 -> Pitch PID controller/1(enable)
  "estimated measures "/1 -> Pitch PID controller/3("estimated measures ")
  references/1 -> Pitch PID controller/2(references)
  Pitch PID controller/1(M) -> M/1  "M_pid"

== system mixTest123/controller/turning controller/roll_controller ==
  enable : Inport
  references : Inport  Port=2
  "estimated measures " : Inport  Port=3
  Roll PID controller : Subsystem
  K : Outport
  wires:
  "estimated measures "/1 -> Roll PID controller/3("estimated measures ")
  Roll PID controller/1(K) -> K/1  "K_pid"
  references/1 -> Roll PID controller/2(references)
  enable/1 -> Roll PID controller/1(enable)

== system mixTest123/controller/turning controller/surge_controller ==
  enable : Inport
  references : Inport  Port=2
  "estimated measures " : Inport  Port=3
  Surge PID controller : Subsystem
  X : Outport
  wires:
  references/1 -> Surge PID controller/2(ref)
  "estimated measures "/1 -> Surge PID controller/3(est_meas)
  Surge PID controller/1(X) -> X/1  "X_pid"
  enable/1 -> Surge PID controller/1(enable)

== system mixTest123/controller/turning controller/sway_controller ==
  enable : Inport
  references : Inport  Port=2
  "estimated measures " : Inport  Port=3
  Sway PID controller : Subsystem
  Y : Outport
  wires:
  enable/1 -> Sway PID controller/1(enable)
  "estimated measures "/1 -> Sway PID controller/3("estimated measures ")
  references/1 -> Sway PID controller/2(references)
  Sway PID controller/1(Y) -> Y/1  "Y_pid"
